simulink model "dPendDisEKF"  (Simulink 7.0)
settings: Solver=ode4  StartTime=0.0  StopTime=10  FixedStep=ts  RelTol=1e-3
InitFcn:
  | %dPendInit;
undefined symbols (not defined in the file): a, accel, B, b, c1, c2, d, evalJacobian, evalJacobMesr, g, l1, m1, m2, magnitude, p, P0, Qe, r1, r2, Re, ts, X0, x_0
libraries: simulink x4
settings Model: Creator=raje_ra  LastModifiedBy=raje_ra  BufferReuse=off
settings OptimizationCC: OptimizeBlockIOStorage=off  BufferReuse=off  ExpressionFolding=off  LocalBlockOutputs=off

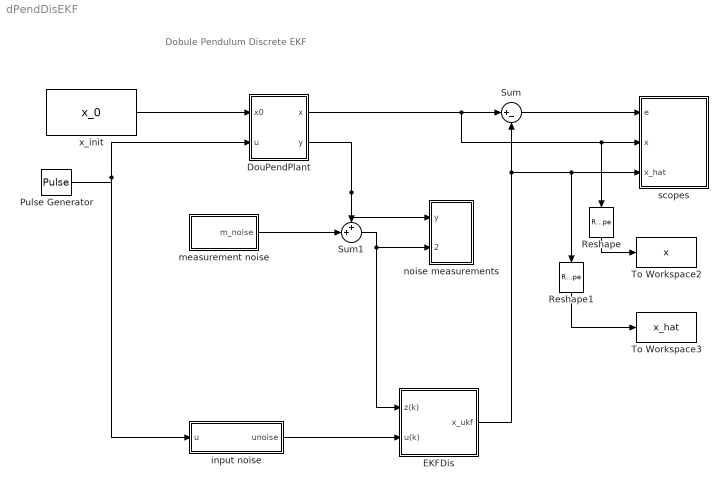
== system dPendDisEKF ==
  note: Dobule Pendulum Discrete EKF
  DouPendPlant : Subsystem
  EKFDis : Subsystem
  Pulse Generator : DiscretePulseGenerator  PulseType=Time based  Amplitude=0.01  Period=1  PulseWidth=50
  Reshape : Reshape  Orientation=down
  Reshape1 : Reshape  Orientation=down
  Sum : Sum  Inputs=|+-  OutDataType=sfix(16)  OutScaling=2^0
  Sum1 : Sum  Inputs=++|  OutDataType=sfix(16)  OutScaling=2^0
  To Workspace2 : ToWorkspace  VariableName=x  SampleTime=-1  SaveFormat=Structure With Time
  To Workspace3 : ToWorkspace  VariableName=x_hat  SampleTime=-1  SaveFormat=Structure With Time
  input noise : Subsystem
  measurement noise : Subsystem
  noise measurements : Subsystem
  scopes : Subsystem
  x_init : Constant  Value=x_0  VectorParams1D=off  OutDataType=sfix(16)  OutScaling=2^0
  wires:
  x_init/1 -> DouPendPlant/1(x0)
  DouPendPlant/1(x) -> Sum/1, scopes/2(x), Reshape/1
  EKFDis/1(x_ukf) -> Sum/2, scopes/3(x_hat), Reshape1/1
  Sum/1 -> scopes/1(e)
  Pulse Generator/1 -> DouPendPlant/2(u), input noise/1(u)
  DouPendPlant/2(y) -> Sum1/1, noise measurements/1(y)
  Sum1/1 -> EKFDis/1(z(k)), noise measurements/2(ynoise)
  measurement noise/1(m_noise) -> Sum1/2
  input noise/1(unoise) -> EKFDis/2(u(k))
  Reshape/1 -> To Workspace2/1
  Reshape1/1 -> To Workspace3/1

== system dPendDisEKF/DouPendPlant ==
  x0 : Inport
  u : Inport  Port=2
  F(x) : Subsystem
  Integrator1 : Integrator  InitialConditionSource=external  InitialCondition=[pi/3,-pi/3]'
  Measurements : Subsystem
  x : Outport  OutDataType=sfix(16)  OutScaling=2^0
  y : Outport  Port=2  OutDataType=sfix(16)  OutScaling=2^0
  wires:
  Measurements/1(y) -> y/1
  x0/1 -> Integrator1/2
  Integrator1/1 -> Measurements/1(x), F(x)/1(x), x/1  "x"
  F(x)/1(x_dot) -> Integrator1/1
  u/1 -> F(x)/2(u), Measurements/2(u)

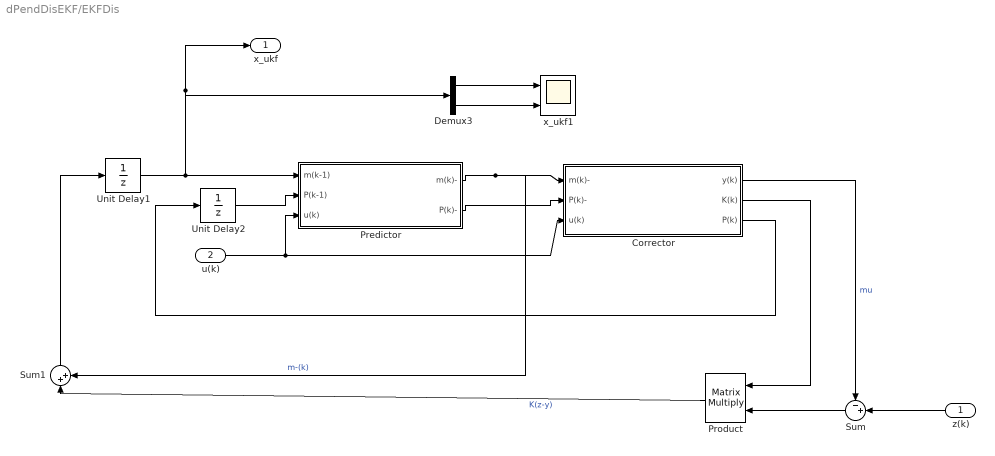
== system dPendDisEKF/EKFDis ==
  z(k) : Inport  Orientation=left
  u(k) : Inport  Port=2
  Corrector : Subsystem
  Demux3 : Demux  Outputs=2
  Predictor : Subsystem
  Product : Product  Orientation=left  Multiplication=Matrix(*)  OutDataType=sfix(16)  OutScaling=2^0  RndMeth=Zero
  Sum : Sum  Orientation=left  Inputs=-+|  OutDataType=sfix(16)  OutScaling=2^0
  Sum1 : Sum  Orientation=up  Inputs=|++  OutDataType=sfix(16)  OutScaling=2^0
  Unit Delay1 : UnitDelay  X0=X0  SampleTime=-1
  Unit Delay2 : UnitDelay  X0=P0  SampleTime=-1
  x_ukf1 : Scope  NumInputPorts=2
      settings: TimeRange=30  YMin=-15~-10  YMax=15~50  SaveName=ScopeData2
  x_ukf : Outport  OutDataType=sfix(16)  OutScaling=2^0
  wires:
  Corrector/3(P(k)) -> Unit Delay2/1
  Unit Delay2/1 -> Predictor/2(P(k-1))
  Product/1 -> Sum1/1  "K(z-y)"
  Sum/1 -> Product/2
  z(k)/1 -> Sum/2
  Corrector/2(K(k)) -> Product/1
  Corrector/1(y(k)) -> Sum/1  "mu"
  Predictor/2(P(k)-) -> Corrector/2(P(k)-)
  Predictor/1(m(k)-) -> Sum1/2, Corrector/1(m(k)-)  "m-(k)"
  Unit Delay1/1 -> Predictor/1(m(k-1)), x_ukf/1, Demux3/1
  Sum1/1 -> Unit Delay1/1
  Demux3/2 -> x_ukf1/2
  Demux3/1 -> x_ukf1/1
  u(k)/1 -> Predictor/3(u(k)), Corrector/3(u(k))

== system dPendDisEKF/input noise ==
  u : Inport
  Band-Limited White Noise : simulink/Sources/Band-Limited White Noise  SystemSampleTime=-1  Cov=[1e-6]  Ts=ts  seed=[23341]
  Sum2 : Sum  Inputs=++|  OutDataType=sfix(16)  OutScaling=2^0
  To Workspace2 : ToWorkspace  VariableName=Q_in  SampleTime=-1  SaveFormat=Array
  unoise : Outport
  wires:
  Band-Limited White Noise/1 -> Sum2/1, To Workspace2/1
  u/1 -> Sum2/2
  Sum2/1 -> unoise/1

== system dPendDisEKF/measurement noise ==
  Band-Limited White Noise - gyro : simulink/Sources/Band-Limited White Noise  SystemSampleTime=-1  Cov=[1e-7]  Ts=ts  seed=[23341]
  Band-Limited White Noise- q,dq : simulink/Sources/Band-Limited White Noise  SystemSampleTime=-1  Cov=[1e-9]  Ts=ts  seed=[23341]
  Band-Limited White Noise-IMU : simulink/Sources/Band-Limited White Noise  SystemSampleTime=-1  Cov=[1e-5]  Ts=ts  seed=[23341]
  Mux : Mux  Inputs=5
  To Workspace : ToWorkspace  VariableName=R_in  SampleTime=-1  SaveFormat=Array
  m_noise : Outport
  wires:
  Band-Limited White Noise- q,dq/1 -> Mux/1, Mux/2
  Mux/1 -> m_noise/1, To Workspace/1
  Band-Limited White Noise - gyro/1 -> Mux/3
  Band-Limited White Noise-IMU/1 -> Mux/4, Mux/5

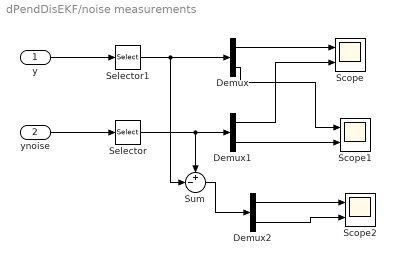
== system dPendDisEKF/noise measurements ==
  y : Inport
  ynoise : Inport  Port=2
  Demux : Demux  Outputs=2
  Demux1 : Demux  Outputs=2
  Demux2 : Demux  Outputs=2
  Scope : Scope  NumInputPorts=2
      settings: YMin=-60~-60  YMax=180~180
  Scope1 : Scope  NumInputPorts=2
      settings: YMin=-60~-60  YMax=180~180  SaveName=ScopeData5
  Scope2 : Scope  NumInputPorts=2
      settings: YMin=-60~-60  YMax=180~180  SaveName=ScopeData6
  Selector : Selector  InputPortWidth=5  IndexOptions=Index vector (dialog)  Indices=[4,5]  OutputSizes=1
  Selector1 : Selector  InputPortWidth=5  IndexOptions=Index vector (dialog)  Indices=[4,5]  OutputSizes=1
  Sum : Sum  Inputs=+-|  OutDataType=sfix(16)  OutScaling=2^0
  wires:
  y/1 -> Selector1/1
  ynoise/1 -> Selector/1
  Selector1/1 -> Demux/1, Sum/2
  Selector/1 -> Demux1/1, Sum/1
  Sum/1 -> Demux2/1
  Demux/1 -> Scope/1
  Demux1/1 -> Scope/2
  Demux/2 -> Scope1/1
  Demux1/2 -> Scope1/2
  Demux2/1 -> Scope2/1
  Demux2/2 -> Scope2/2

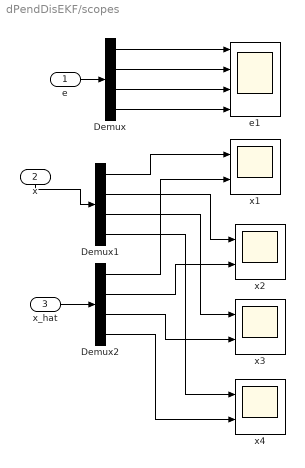
== system dPendDisEKF/scopes ==
  e : Inport
  x : Inport  Orientation=down  Port=2
  x_hat : Inport  Port=3
  Demux : Demux
  Demux1 : Demux
  Demux2 : Demux
  e1 : Scope  NumInputPorts=4
      settings: TickLabels=on  YMin=-30~-20~-120~-17.5  YMax=80~27.5~20~25
  x{1..4} (4 alike) : Scope  NumInputPorts=2
      x1 settings: TickLabels=on  YMin=-5~-5  YMax=14~22.5  SaveName=ScopeData3
      x2 settings: TickLabels=on  YMin=-11~-11  YMax=11~11  SaveName=ScopeData4
      x3 settings: TickLabels=on  YMin=-10~-10  YMax=27.5~27.5  SaveName=ScopeData7
      x4 settings: TickLabels=on  YMin=-40~-40  YMax=35~35  SaveName=ScopeData8
  wires:
  e/1 -> Demux/1
  x_hat/1 -> Demux2/1
  x/1 -> Demux1/1
  Demux2/4 -> x4/2
  Demux1/4 -> x4/1
  Demux2/3 -> x3/2
  Demux1/3 -> x3/1
  Demux2/2 -> x2/2
  Demux1/2 -> x2/1
  Demux2/1 -> x1/2
  Demux1/1 -> x1/1
  Demux/4 -> e1/4
  Demux/3 -> e1/3
  Demux/2 -> e1/2
  Demux/1 -> e1/1

== system dPendDisEKF/DouPendPlant/F(x) ==
  x : Inport
  u : Inport  Port=2
  Add : Sum  Inputs=+++  OutDataType=sfix(16)  OutScaling=2^-10
  Divide : Product  Inputs=/*  Multiplication=Matrix(*)  OutDataType=sfix(16)  OutScaling=2^-10
  Gain : Gain  Gain=diag([0,c1,0,c2])  Multiplication=Matrix(K*u)  ParameterDataType=sfix(16)  ParameterScaling=2^0  OutDataType=sfix(16)  OutScaling=2^0
  Gain1 : Gain  Gain=B  ParameterDataType=sfix(16)  ParameterScaling=2^0  OutDataType=sfix(16)  OutScaling=2^0
  M matrix : Subsystem
  h+g : Subsystem
  x_dot : Outport
  wires:
  Divide/1 -> x_dot/1
  M matrix/1(M) -> Divide/1
  Gain1/1 -> Add/3
  Add/1 -> Divide/2
  u/1 -> Gain1/1
  Gain/1 -> Add/2
  h+g/1(-(h+g)) -> Add/1
  x/1 -> Gain/1, h+g/1(x), M matrix/1(x)

== system dPendDisEKF/DouPendPlant/Measurements ==
  x : Inport
  u : Inport  Port=2
  Display : Display
  IMU : Subsystem
  Mux : Mux  Inputs=3
  Selector1 : Selector  InputPortWidth=4  IndexOptions=Index vector (dialog)  Indices=[3 4]  OutputSizes=1
  Selector2 : Selector  InputPortWidth=4  IndexOptions=Index vector (dialog)  Indices=[2 4]  OutputSizes=1
  Sum of Elements : Sum  Inputs=+  OutDataType=sfix(16)  OutScaling=2^-10
  y : Outport  OutDataType=sfix(16)  OutScaling=2^0
  wires:
  x/1 -> Selector1/1, Selector2/1, IMU/1(m(k)-)
  Selector1/1 -> Mux/1
  Mux/1 -> y/1, Display/1
  Selector2/1 -> Sum of Elements/1
  Sum of Elements/1 -> Mux/2  "(dq_1+dq_2)"
  u/1 -> IMU/2(u(k))
  IMU/1(acc) -> Mux/3

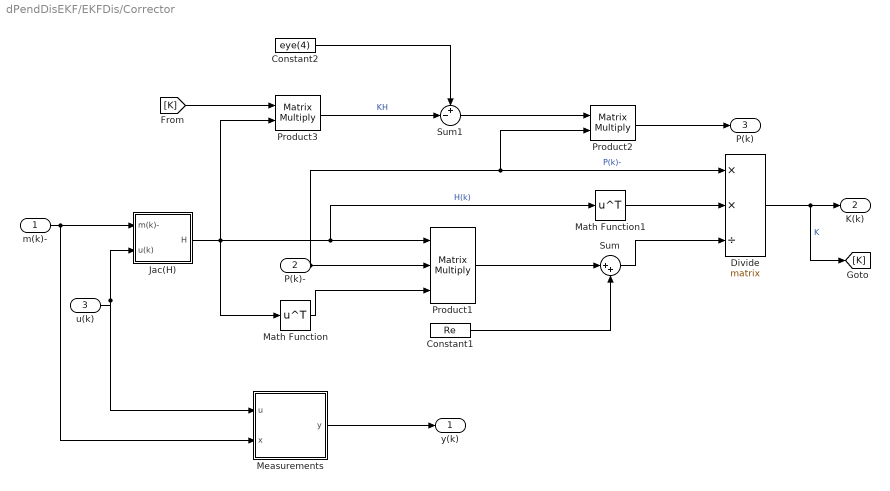
== system dPendDisEKF/EKFDis/Corrector ==
  m(k)- : Inport
  P(k)- : Inport  Port=2
  u(k) : Inport  Port=3
  Constant1 : Constant  Value=Re  OutDataType=sfix(16)  OutScaling=2^0
  Constant2 : Constant  Value=eye(4)  VectorParams1D=off  OutDataType=sfix(16)  OutScaling=2^0
  Divide : Product  Inputs=**/  Multiplication=Matrix(*)  OutDataType=sfix(16)  OutScaling=2^-10
  Jac(H) : Subsystem
  Math Function : Math  Operator=transpose  OutDataType=sfix(16)  OutScaling=2^0  SaturateOnIntegerOverflow=on
  Math Function1 : Math  Operator=transpose  OutDataType=sfix(16)  OutScaling=2^0  SaturateOnIntegerOverflow=on
  Measurements : Subsystem
  Product1 : Product  Inputs=3  Multiplication=Matrix(*)  OutDataType=sfix(16)  OutScaling=2^0  RndMeth=Zero
  Product2 : Product  Multiplication=Matrix(*)  OutDataType=sfix(16)  OutScaling=2^0  RndMeth=Zero
  Product3 : Product  Multiplication=Matrix(*)  OutDataType=sfix(16)  OutScaling=2^0  RndMeth=Zero
  Sum : Sum  Inputs=|++  OutDataType=sfix(16)  OutScaling=2^0
  Sum1 : Sum  Inputs=+-|  OutDataType=sfix(16)  OutScaling=2^0
  y(k) : Outport
  K(k) : Outport  Port=2
  P(k) : Outport  Port=3
  wires:
  Constant1/1 -> Sum/2
  Product1/1 -> Sum/1
  m(k)-/1 -> Jac(H)/1(m(k)-), Measurements/2(x)
  u(k)/1 -> Jac(H)/2(u(k)), Measurements/1(u)
  Jac(H)/1(H) -> Math Function/1, Product3/2, Product1/1, Math Function1/1  "H(k)"
  P(k)-/1 -> Product1/2, Divide/1, Product2/2  "P(k)-"
  Math Function/1 -> Product1/3
  Sum/1 -> Divide/3
  Divide/1 -> K(k)/1, [K]  "K"
  [K] -> Product3/1
  Constant2/1 -> Sum1/1
  Product3/1 -> Sum1/2  "KH"
  Sum1/1 -> Product2/1
  Product2/1 -> P(k)/1
  Measurements/1(y) -> y(k)/1
  Math Function1/1 -> Divide/2

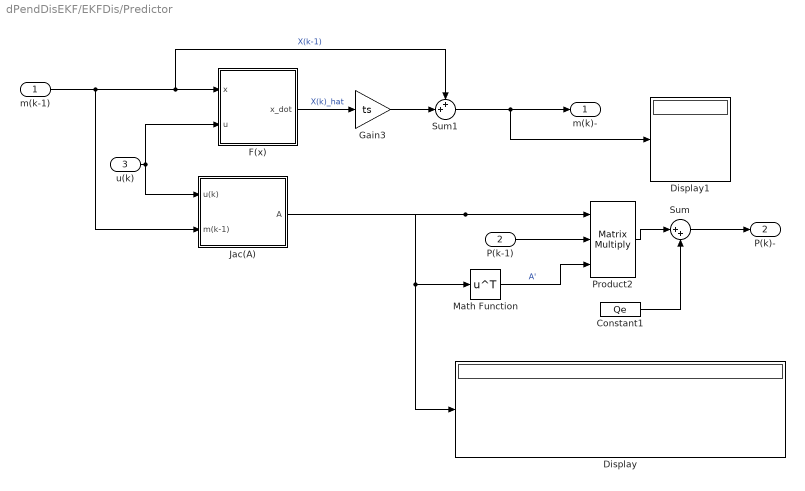
== system dPendDisEKF/EKFDis/Predictor ==
  m(k-1) : Inport
  P(k-1) : Inport  Port=2
  u(k) : Inport  Port=3
  Constant1 : Constant  Value=Qe  OutDataType=sfix(16)  OutScaling=2^0
  Display : Display
  Display1 : Display
  F(x) : Subsystem
  Gain3 : Gain  Gain=ts  ParameterDataType=sfix(16)  ParameterScaling=2^0  OutDataType=sfix(16)  OutScaling=2^0
  Jac(A) : Subsystem
  Math Function : Math  Operator=transpose  OutDataType=sfix(16)  OutScaling=2^0  SaturateOnIntegerOverflow=on
  Product2 : Product  Inputs=3  Multiplication=Matrix(*)  OutDataType=sfix(16)  OutScaling=2^0  RndMeth=Zero
  Sum : Sum  Inputs=|++  OutDataType=sfix(16)  OutScaling=2^0
  Sum1 : Sum  Inputs=++|  OutDataType=sfix(16)  OutScaling=2^0
  m(k)- : Outport
  P(k)- : Outport  Port=2
  wires:
  Sum/1 -> P(k)-/1
  Constant1/1 -> Sum/2
  Product2/1 -> Sum/1
  m(k-1)/1 -> Jac(A)/2(m(k-1)), F(x)/1(x), Sum1/1  "X(k-1)"
  u(k)/1 -> Jac(A)/1(u(k)), F(x)/2(u)
  F(x)/1(x_dot) -> Gain3/1  "X(k)_hat"
  Jac(A)/1(A) -> Product2/1, Math Function/1, Display/1
  P(k-1)/1 -> Product2/2
  Math Function/1 -> Product2/3  "A'"
  Gain3/1 -> Sum1/2
  Sum1/1 -> m(k)-/1, Display1/1

== system dPendDisEKF/DouPendPlant/F(x)/M matrix ==
  x : Inport
  M1 : Constant  Value=[1,0,0,0]  VectorParams1D=off  OutDataType=sfix(16)  OutScaling=2^0
  M2 : Subsystem
  M3 : Constant  Value=[0,0,1,0]  VectorParams1D=off  OutDataType=sfix(16)  OutScaling=2^0
  M4 : Subsystem
  Matrix Concatenate : Concatenate  NumInputs=4  Mode=Multidimensional array
  Selector : Selector  InputPortWidth=4  IndexOptions=Index vector (dialog)  Indices=[3]  OutputSizes=1
  M : Outport
  wires:
  Matrix Concatenate/1 -> M/1
  x/1 -> Selector/1
  M4/1(Out) -> Matrix Concatenate/4
  M3/1 -> Matrix Concatenate/3
  M2/1(Out1) -> Matrix Concatenate/2
  M1/1 -> Matrix Concatenate/1
  Selector/1 -> M4/1(x3), M2/1(x3)  "x3"

== system dPendDisEKF/DouPendPlant/F(x)/h+g ==
  x : Inport
  Selector : Selector  InputPortWidth=4  IndexOptions=Index vector (dialog)  Indices=[2]  OutputSizes=1
  Selector1 : Selector  InputPortWidth=4  IndexOptions=Index vector (dialog)  Indices=[4]  OutputSizes=1
  Vector Concatenate : Concatenate  NumInputs=4  Mode=Vector
  h+g(2) : Subsystem
  h+g(4) : Subsystem
  -(h+g) : Outport
  wires:
  Vector Concatenate/1 -> -(h+g)/1
  h+g(4)/1(-F(2)) -> Vector Concatenate/4
  Selector1/1 -> Vector Concatenate/3
  h+g(2)/1(-F(1)) -> Vector Concatenate/2
  Selector/1 -> Vector Concatenate/1  "x2"
  x/1 -> h+g(4)/1(x), Selector1/1, h+g(2)/1(x), Selector/1

== system dPendDisEKF/DouPendPlant/Measurements/IMU ==
  m(k)- : Inport
  u(k) : Inport  Port=2
  Mux : Mux  Inputs=2
  Transpose : Math  Operator=transpose  OutDataType=sfix(16)  OutScaling=2^0  SaturateOnIntegerOverflow=on
  acceleration : MATLABFcn  MATLABFcn=accel(u,p)  Output1D=off
  acc : Outport
  wires:
  Mux/1 -> Transpose/1
  Transpose/1 -> acceleration/1
  m(k)-/1 -> Mux/1
  acceleration/1 -> acc/1  "acc"
  u(k)/1 -> Mux/2

== system dPendDisEKF/EKFDis/Corrector/Jac(H) ==
  m(k)- : Inport
  u(k) : Inport  Port=2
  Display : Display
  Display1 : Display
  Jacob Mesr : MATLABFcn  MATLABFcn=evalJacobMesr(u,p)  Output1D=off
  Mux : Mux  Inputs=2
  Transpose : Math  Operator=transpose  OutDataType=sfix(16)  OutScaling=2^0  SaturateOnIntegerOverflow=on
  H : Outport
  wires:
  Mux/1 -> Transpose/1, Display1/1
  Transpose/1 -> Jacob Mesr/1
  m(k)-/1 -> Mux/1
  Jacob Mesr/1 -> H/1, Display/1  "h"
  u(k)/1 -> Mux/2

== system dPendDisEKF/EKFDis/Corrector/Measurements ==
  u : Inport
  x : Inport  Port=2
  IMU : Subsystem
  Mux : Mux  Inputs=3
  Selector1 : Selector  InputPortWidth=4  IndexOptions=Index vector (dialog)  Indices=[3 4]  OutputSizes=1
  Selector2 : Selector  InputPortWidth=4  IndexOptions=Index vector (dialog)  Indices=[2 4]  OutputSizes=1
  Sum of Elements : Sum  Inputs=+  OutDataType=sfix(16)  OutScaling=2^-10
  y : Outport  OutDataType=sfix(16)  OutScaling=2^0
  wires:
  x/1 -> Selector1/1, Selector2/1, IMU/1(m(k)-)
  Selector1/1 -> Mux/1
  Mux/1 -> y/1
  Selector2/1 -> Sum of Elements/1
  Sum of Elements/1 -> Mux/2  "(dq_1+dq_2)"
  u/1 -> IMU/2(u(k))
  IMU/1(acc) -> Mux/3

== system dPendDisEKF/EKFDis/Predictor/F(x) ==
  x : Inport
  u : Inport  Port=2
  Add : Sum  Inputs=+++  OutDataType=sfix(16)  OutScaling=2^-10
  Divide : Product  Inputs=/*  Multiplication=Matrix(*)  OutDataType=sfix(16)  OutScaling=2^-10
  Gain : Gain  Gain=diag([0,c1,0,c2])  Multiplication=Matrix(K*u)  ParameterDataType=sfix(16)  ParameterScaling=2^0  OutDataType=sfix(16)  OutScaling=2^0
  Gain1 : Gain  Gain=B  ParameterDataType=sfix(16)  ParameterScaling=2^0  OutDataType=sfix(16)  OutScaling=2^0
  M matrix : Subsystem
  h+g : Subsystem
  x_dot : Outport
  wires:
  Divide/1 -> x_dot/1
  M matrix/1(M) -> Divide/1
  Gain1/1 -> Add/3
  Add/1 -> Divide/2
  u/1 -> Gain1/1
  Gain/1 -> Add/2
  h+g/1(-(h+g)) -> Add/1
  x/1 -> h+g/1(x), Gain/1, M matrix/1(x)

== system dPendDisEKF/EKFDis/Predictor/Jac(A) ==
  u(k) : Inport
  m(k-1) : Inport  Port=2
  Display : Display
  Display1 : Display
  MATLAB Fcn : MATLABFcn  MATLABFcn=evalJacobian(u,p)  Output1D=off
  Math Function1 : Math  Operator=transpose  OutDataType=sfix(16)  OutScaling=2^0  SaturateOnIntegerOverflow=on
  Mux : Mux  Inputs=2
  A : Outport
  wires:
  Math Function1/1 -> MATLAB Fcn/1, Display1/1
  MATLAB Fcn/1 -> A/1, Display/1  "A"
  m(k-1)/1 -> Mux/1
  u(k)/1 -> Mux/2
  Mux/1 -> Math Function1/1

== system dPendDisEKF/DouPendPlant/F(x)/M matrix/M2 ==
  x3 : Inport
  M21 : Constant  Value=0  VectorParams1D=off  OutDataType=sfix(16)  OutScaling=2^0
  M22 : Subsystem
  M23 : Constant  Value=0  VectorParams1D=off  OutDataType=sfix(16)  OutScaling=2^0
  M24 : Subsystem
  Math Function : Math  Operator=transpose  OutDataType=sfix(16)  OutScaling=2^0  SaturateOnIntegerOverflow=on
  Vector Concatenate : Concatenate  NumInputs=4  Mode=Vector
  Out1 : Outport
  wires:
  Math Function/1 -> Out1/1
  Vector Concatenate/1 -> Math Function/1
  M24/1(M24) -> Vector Concatenate/4
  M23/1 -> Vector Concatenate/3
  M22/1(M22) -> Vector Concatenate/2
  M21/1 -> Vector Concatenate/1
  x3/1 -> M24/1(x3), M22/1(x3)

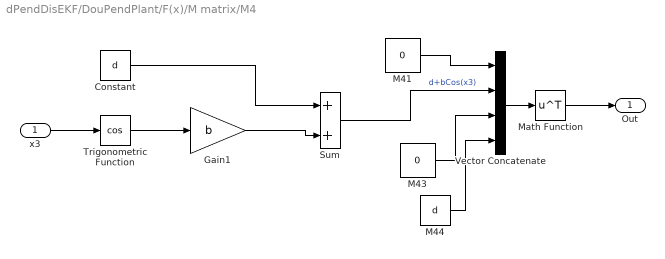
== system dPendDisEKF/DouPendPlant/F(x)/M matrix/M4 ==
  x3 : Inport
  Constant : Constant  Value=d  OutDataType=sfix(16)  OutScaling=2^0
  Gain1 : Gain  Gain=b  ParameterDataType=sfix(16)  ParameterScaling=2^0  OutDataType=sfix(16)  OutScaling=2^0
  M41 : Constant  Value=0  VectorParams1D=off  OutDataType=sfix(16)  OutScaling=2^0
  M43 : Constant  Value=0  VectorParams1D=off  OutDataType=sfix(16)  OutScaling=2^0
  M44 : Constant  Value=d  OutDataType=sfix(16)  OutScaling=2^0
  Math Function : Math  Operator=transpose  OutDataType=sfix(16)  OutScaling=2^0  SaturateOnIntegerOverflow=on
  Sum : Sum  OutDataType=sfix(16)  OutScaling=2^0
  Trigonometric Function : Trigonometry  Operator=cos
  Vector Concatenate : Concatenate  NumInputs=4  Mode=Vector
  Out : Outport
  wires:
  Constant/1 -> Sum/1
  Math Function/1 -> Out/1
  Vector Concatenate/1 -> Math Function/1
  M43/1 -> Vector Concatenate/3
  M44/1 -> Vector Concatenate/4
  Sum/1 -> Vector Concatenate/2  "d+bCos(x3)"
  M41/1 -> Vector Concatenate/1
  Trigonometric Function/1 -> Gain1/1
  Gain1/1 -> Sum/2
  x3/1 -> Trigonometric Function/1

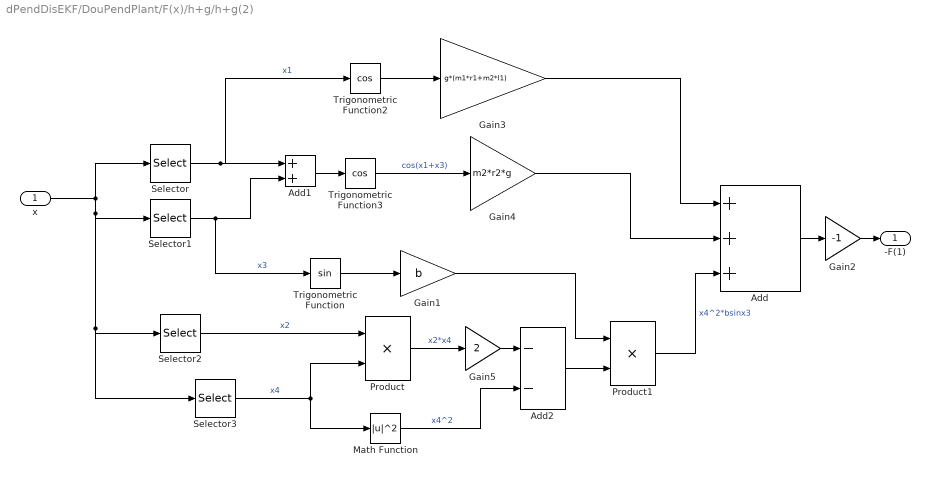
== system dPendDisEKF/DouPendPlant/F(x)/h+g/h+g(2) ==
  x : Inport
  Add : Sum  Inputs=+++  OutDataType=sfix(16)  OutScaling=2^-10
  Add1 : Sum  OutDataType=sfix(16)  OutScaling=2^-10
  Add2 : Sum  Inputs=--  OutDataType=sfix(16)  OutScaling=2^-10
  Gain1 : Gain  Gain=b  ParameterDataType=sfix(16)  ParameterScaling=2^0  OutDataType=sfix(16)  OutScaling=2^0
  Gain2 : Gain  Gain=-1  ParameterDataType=sfix(16)  ParameterScaling=2^0  OutDataType=sfix(16)  OutScaling=2^0
  Gain3 : Gain  Gain=g*(m1*r1+m2*l1)  ParameterDataType=sfix(16)  ParameterScaling=2^0  OutDataType=sfix(16)  OutScaling=2^0
  Gain4 : Gain  Gain=m2*r2*g  ParameterDataType=sfix(16)  ParameterScaling=2^0  OutDataType=sfix(16)  OutScaling=2^0
  Gain5 : Gain  Gain=2  ParameterDataType=sfix(16)  ParameterScaling=2^0  OutDataType=sfix(16)  OutScaling=2^0
  Math Function : Math  Operator=magnitude^2  OutDataType=sfix(16)  OutScaling=2^0  SaturateOnIntegerOverflow=on
  Product : Product  OutDataType=sfix(16)  OutScaling=2^0  RndMeth=Zero
  Product1 : Product  OutDataType=sfix(16)  OutScaling=2^0  RndMeth=Zero
  Selector : Selector  InputPortWidth=4  IndexOptions=Index vector (dialog)  Indices=[1]  OutputSizes=1
  Selector1 : Selector  InputPortWidth=4  IndexOptions=Index vector (dialog)  Indices=[3]  OutputSizes=1
  Selector2 : Selector  InputPortWidth=4  IndexOptions=Index vector (dialog)  Indices=[2]  OutputSizes=1
  Selector3 : Selector  InputPortWidth=4  IndexOptions=Index vector (dialog)  Indices=[4]  OutputSizes=1
  Trigonometric Function : Trigonometry
  Trigonometric Function2 : Trigonometry  Operator=cos
  Trigonometric Function3 : Trigonometry  Operator=cos
  -F(1) : Outport  OutDataType=sfix(16)  OutScaling=2^0
  wires:
  Gain2/1 -> -F(1)/1
  Gain1/1 -> Product1/1
  Add2/1 -> Product1/2
  Gain5/1 -> Add2/1
  Product/1 -> Gain5/1  "x2*x4"
  Math Function/1 -> Add2/2  "x4^2"
  Selector2/1 -> Product/1  "x2"
  Selector3/1 -> Math Function/1, Product/2  "x4"
  x/1 -> Selector3/1, Selector2/1, Selector1/1, Selector/1
  Add/1 -> Gain2/1
  Product1/1 -> Add/3  "x4^2*bsinx3"
  Gain4/1 -> Add/2
  Add1/1 -> Trigonometric Function3/1
  Trigonometric Function3/1 -> Gain4/1  "cos(x1+x3)"
  Gain3/1 -> Add/1
  Trigonometric Function2/1 -> Gain3/1
  Selector/1 -> Trigonometric Function2/1, Add1/1  "x1"
  Selector1/1 -> Trigonometric Function/1, Add1/2  "x3"
  Trigonometric Function/1 -> Gain1/1

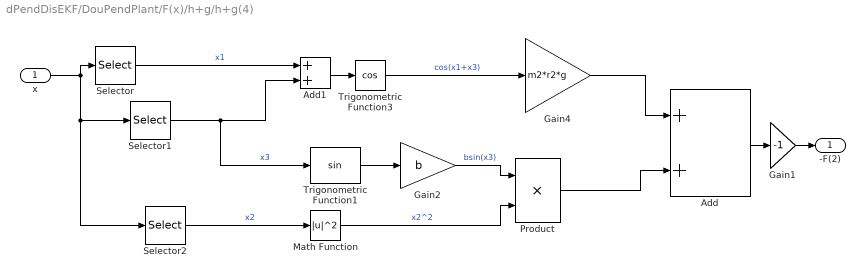
== system dPendDisEKF/DouPendPlant/F(x)/h+g/h+g(4) ==
  x : Inport
  Add : Sum  OutDataType=sfix(16)  OutScaling=2^-10
  Add1 : Sum  OutDataType=sfix(16)  OutScaling=2^-10
  Gain1 : Gain  Gain=-1  ParameterDataType=sfix(16)  ParameterScaling=2^0  OutDataType=sfix(16)  OutScaling=2^0
  Gain2 : Gain  Gain=b  ParameterDataType=sfix(16)  ParameterScaling=2^0  OutDataType=sfix(16)  OutScaling=2^0
  Gain4 : Gain  Gain=m2*r2*g  ParameterDataType=sfix(16)  ParameterScaling=2^0  OutDataType=sfix(16)  OutScaling=2^0
  Math Function : Math  Operator=magnitude^2  OutDataType=sfix(16)  OutScaling=2^0  SaturateOnIntegerOverflow=on
  Product : Product  OutDataType=sfix(16)  OutScaling=2^0  RndMeth=Zero
  Selector : Selector  InputPortWidth=4  IndexOptions=Index vector (dialog)  Indices=[1]  OutputSizes=1
  Selector1 : Selector  InputPortWidth=4  IndexOptions=Index vector (dialog)  Indices=[3]  OutputSizes=1
  Selector2 : Selector  InputPortWidth=4  IndexOptions=Index vector (dialog)  Indices=[2]  OutputSizes=1
  Trigonometric Function1 : Trigonometry
  Trigonometric Function3 : Trigonometry  Operator=cos
  -F(2) : Outport  OutDataType=sfix(16)  OutScaling=2^0
  wires:
  Gain1/1 -> -F(2)/1
  Math Function/1 -> Product/2  "x2^2"
  Gain2/1 -> Product/1  "bsin(x3)"
  Add/1 -> Gain1/1
  Add1/1 -> Trigonometric Function3/1
  Trigonometric Function3/1 -> Gain4/1  "cos(x1+x3)"
  Selector/1 -> Add1/1  "x1"
  Selector1/1 -> Add1/2, Trigonometric Function1/1  "x3"
  Trigonometric Function1/1 -> Gain2/1
  x/1 -> Selector2/1, Selector1/1, Selector/1
  Gain4/1 -> Add/1
  Product/1 -> Add/2
  Selector2/1 -> Math Function/1  "x2"

== system dPendDisEKF/EKFDis/Corrector/Measurements/IMU ==
  m(k)- : Inport
  u(k) : Inport  Port=2
  Mux : Mux  Inputs=2
  Transpose : Math  Operator=transpose  OutDataType=sfix(16)  OutScaling=2^0  SaturateOnIntegerOverflow=on
  accleration : MATLABFcn  MATLABFcn=accel(u,p)  Output1D=off
  acc : Outport
  wires:
  Mux/1 -> Transpose/1
  Transpose/1 -> accleration/1
  m(k)-/1 -> Mux/1
  accleration/1 -> acc/1  "acc"
  u(k)/1 -> Mux/2

== system dPendDisEKF/EKFDis/Predictor/F(x)/M matrix ==
  x : Inport
  M1 : Constant  Value=[1,0,0,0]  VectorParams1D=off  OutDataType=sfix(16)  OutScaling=2^0
  M2 : Subsystem
  M3 : Constant  Value=[0,0,1,0]  VectorParams1D=off  OutDataType=sfix(16)  OutScaling=2^0
  M4 : Subsystem
  Matrix Concatenate : Concatenate  NumInputs=4  Mode=Multidimensional array
  Selector : Selector  InputPortWidth=4  IndexOptions=Index vector (dialog)  Indices=[3]  OutputSizes=1
  M : Outport
  wires:
  Matrix Concatenate/1 -> M/1
  x/1 -> Selector/1
  M4/1(Out) -> Matrix Concatenate/4
  M3/1 -> Matrix Concatenate/3
  M2/1(Out1) -> Matrix Concatenate/2
  M1/1 -> Matrix Concatenate/1
  Selector/1 -> M4/1(x3), M2/1(x3)  "x3"

== system dPendDisEKF/EKFDis/Predictor/F(x)/h+g ==
  x : Inport
  Selector : Selector  InputPortWidth=4  IndexOptions=Index vector (dialog)  Indices=[2]  OutputSizes=1
  Selector1 : Selector  InputPortWidth=4  IndexOptions=Index vector (dialog)  Indices=[4]  OutputSizes=1
  Vector Concatenate : Concatenate  NumInputs=4  Mode=Vector
  h+g(2) : Subsystem
  h+g(4) : Subsystem
  -(h+g) : Outport
  wires:
  Vector Concatenate/1 -> -(h+g)/1
  h+g(4)/1(-F(2)) -> Vector Concatenate/4
  Selector1/1 -> Vector Concatenate/3
  h+g(2)/1(-F(1)) -> Vector Concatenate/2
  Selector/1 -> Vector Concatenate/1  "x2"
  x/1 -> h+g(4)/1(x), Selector1/1, h+g(2)/1(x), Selector/1

== system dPendDisEKF/DouPendPlant/F(x)/M matrix/M2/M22 ==
  x3 : Inport
  Constant : Constant  Value=a  OutDataType=sfix(16)  OutScaling=2^0
  Gain1 : Gain  Gain=2*b  ParameterDataType=sfix(16)  ParameterScaling=2^0  OutDataType=sfix(16)  OutScaling=2^0
  Sum : Sum  OutDataType=sfix(16)  OutScaling=2^0
  Trigonometric Function : Trigonometry  Operator=cos
  M22 : Outport
  wires:
  Constant/1 -> Sum/1
  Trigonometric Function/1 -> Gain1/1
  Gain1/1 -> Sum/2
  Sum/1 -> M22/1  "a+2bCos(x3)"
  x3/1 -> Trigonometric Function/1

== system dPendDisEKF/DouPendPlant/F(x)/M matrix/M2/M24 ==
  x3 : Inport
  Constant : Constant  Value=d  OutDataType=sfix(16)  OutScaling=2^0
  Gain1 : Gain  Gain=b  ParameterDataType=sfix(16)  ParameterScaling=2^0  OutDataType=sfix(16)  OutScaling=2^0
  Sum : Sum  OutDataType=sfix(16)  OutScaling=2^0
  Trigonometric Function : Trigonometry  Operator=cos
  M24 : Outport
  wires:
  Constant/1 -> Sum/1
  x3/1 -> Trigonometric Function/1
  Sum/1 -> M24/1  "d+bCos(x3)"
  Gain1/1 -> Sum/2
  Trigonometric Function/1 -> Gain1/1

== system dPendDisEKF/EKFDis/Predictor/F(x)/M matrix/M2 ==
  x3 : Inport
  M21 : Constant  Value=0  VectorParams1D=off  OutDataType=sfix(16)  OutScaling=2^0
  M22 : Subsystem
  M23 : Constant  Value=0  VectorParams1D=off  OutDataType=sfix(16)  OutScaling=2^0
  M24 : Subsystem
  Math Function : Math  Operator=transpose  OutDataType=sfix(16)  OutScaling=2^0  SaturateOnIntegerOverflow=on
  Vector Concatenate : Concatenate  NumInputs=4  Mode=Vector
  Out1 : Outport
  wires:
  Math Function/1 -> Out1/1
  Vector Concatenate/1 -> Math Function/1
  M24/1(M24) -> Vector Concatenate/4
  M23/1 -> Vector Concatenate/3
  M22/1(M22) -> Vector Concatenate/2
  M21/1 -> Vector Concatenate/1
  x3/1 -> M24/1(x3), M22/1(x3)

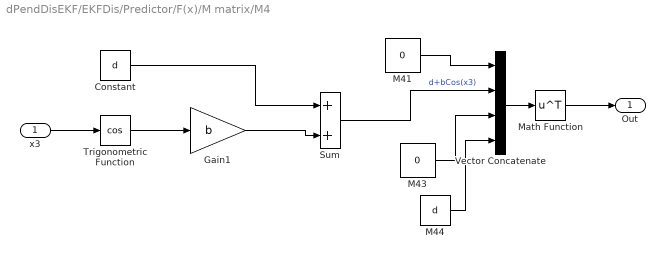
== system dPendDisEKF/EKFDis/Predictor/F(x)/M matrix/M4 ==
  x3 : Inport
  Constant : Constant  Value=d  OutDataType=sfix(16)  OutScaling=2^0
  Gain1 : Gain  Gain=b  ParameterDataType=sfix(16)  ParameterScaling=2^0  OutDataType=sfix(16)  OutScaling=2^0
  M41 : Constant  Value=0  VectorParams1D=off  OutDataType=sfix(16)  OutScaling=2^0
  M43 : Constant  Value=0  VectorParams1D=off  OutDataType=sfix(16)  OutScaling=2^0
  M44 : Constant  Value=d  OutDataType=sfix(16)  OutScaling=2^0
  Math Function : Math  Operator=transpose  OutDataType=sfix(16)  OutScaling=2^0  SaturateOnIntegerOverflow=on
  Sum : Sum  OutDataType=sfix(16)  OutScaling=2^0
  Trigonometric Function : Trigonometry  Operator=cos
  Vector Concatenate : Concatenate  NumInputs=4  Mode=Vector
  Out : Outport
  wires:
  Constant/1 -> Sum/1
  Math Function/1 -> Out/1
  Vector Concatenate/1 -> Math Function/1
  M43/1 -> Vector Concatenate/3
  M44/1 -> Vector Concatenate/4
  Sum/1 -> Vector Concatenate/2  "d+bCos(x3)"
  M41/1 -> Vector Concatenate/1
  Trigonometric Function/1 -> Gain1/1
  Gain1/1 -> Sum/2
  x3/1 -> Trigonometric Function/1

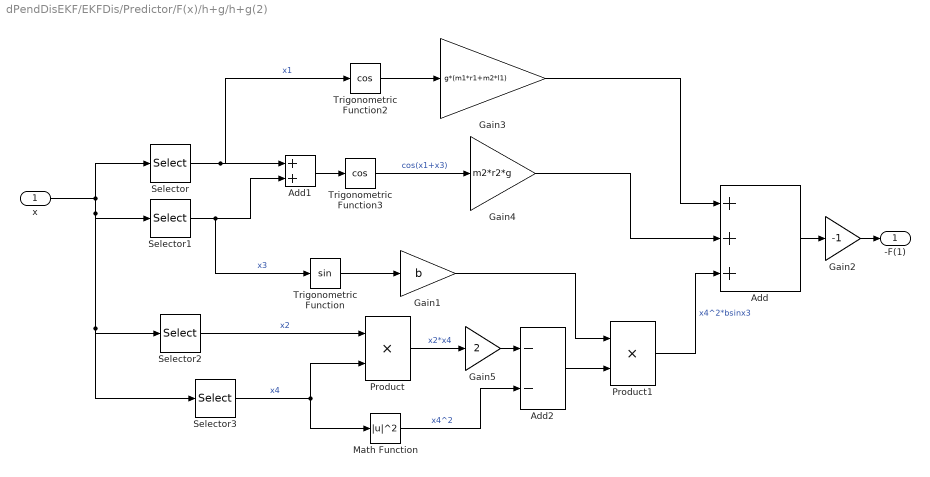
== system dPendDisEKF/EKFDis/Predictor/F(x)/h+g/h+g(2) ==
  x : Inport
  Add : Sum  Inputs=+++  OutDataType=sfix(16)  OutScaling=2^-10
  Add1 : Sum  OutDataType=sfix(16)  OutScaling=2^-10
  Add2 : Sum  Inputs=--  OutDataType=sfix(16)  OutScaling=2^-10
  Gain1 : Gain  Gain=b  ParameterDataType=sfix(16)  ParameterScaling=2^0  OutDataType=sfix(16)  OutScaling=2^0
  Gain2 : Gain  Gain=-1  ParameterDataType=sfix(16)  ParameterScaling=2^0  OutDataType=sfix(16)  OutScaling=2^0
  Gain3 : Gain  Gain=g*(m1*r1+m2*l1)  ParameterDataType=sfix(16)  ParameterScaling=2^0  OutDataType=sfix(16)  OutScaling=2^0
  Gain4 : Gain  Gain=m2*r2*g  ParameterDataType=sfix(16)  ParameterScaling=2^0  OutDataType=sfix(16)  OutScaling=2^0
  Gain5 : Gain  Gain=2  ParameterDataType=sfix(16)  ParameterScaling=2^0  OutDataType=sfix(16)  OutScaling=2^0
  Math Function : Math  Operator=magnitude^2  OutDataType=sfix(16)  OutScaling=2^0  SaturateOnIntegerOverflow=on
  Product : Product  OutDataType=sfix(16)  OutScaling=2^0  RndMeth=Zero
  Product1 : Product  OutDataType=sfix(16)  OutScaling=2^0  RndMeth=Zero
  Selector : Selector  InputPortWidth=4  IndexOptions=Index vector (dialog)  Indices=[1]  OutputSizes=1
  Selector1 : Selector  InputPortWidth=4  IndexOptions=Index vector (dialog)  Indices=[3]  OutputSizes=1
  Selector2 : Selector  InputPortWidth=4  IndexOptions=Index vector (dialog)  Indices=[2]  OutputSizes=1
  Selector3 : Selector  InputPortWidth=4  IndexOptions=Index vector (dialog)  Indices=[4]  OutputSizes=1
  Trigonometric Function : Trigonometry
  Trigonometric Function2 : Trigonometry  Operator=cos
  Trigonometric Function3 : Trigonometry  Operator=cos
  -F(1) : Outport  OutDataType=sfix(16)  OutScaling=2^0
  wires:
  Gain2/1 -> -F(1)/1
  Gain1/1 -> Product1/1
  Add2/1 -> Product1/2
  Gain5/1 -> Add2/1
  Product/1 -> Gain5/1  "x2*x4"
  Math Function/1 -> Add2/2  "x4^2"
  Selector2/1 -> Product/1  "x2"
  Selector3/1 -> Math Function/1, Product/2  "x4"
  x/1 -> Selector3/1, Selector2/1, Selector1/1, Selector/1
  Add/1 -> Gain2/1
  Product1/1 -> Add/3  "x4^2*bsinx3"
  Gain4/1 -> Add/2
  Add1/1 -> Trigonometric Function3/1
  Trigonometric Function3/1 -> Gain4/1  "cos(x1+x3)"
  Gain3/1 -> Add/1
  Trigonometric Function2/1 -> Gain3/1
  Selector/1 -> Trigonometric Function2/1, Add1/1  "x1"
  Selector1/1 -> Trigonometric Function/1, Add1/2  "x3"
  Trigonometric Function/1 -> Gain1/1

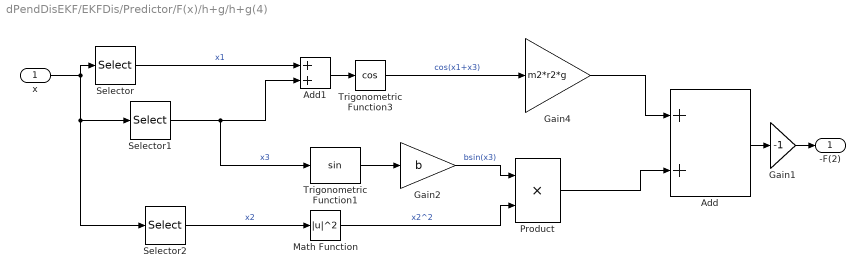
== system dPendDisEKF/EKFDis/Predictor/F(x)/h+g/h+g(4) ==
  x : Inport
  Add : Sum  OutDataType=sfix(16)  OutScaling=2^-10
  Add1 : Sum  OutDataType=sfix(16)  OutScaling=2^-10
  Gain1 : Gain  Gain=-1  ParameterDataType=sfix(16)  ParameterScaling=2^0  OutDataType=sfix(16)  OutScaling=2^0
  Gain2 : Gain  Gain=b  ParameterDataType=sfix(16)  ParameterScaling=2^0  OutDataType=sfix(16)  OutScaling=2^0
  Gain4 : Gain  Gain=m2*r2*g  ParameterDataType=sfix(16)  ParameterScaling=2^0  OutDataType=sfix(16)  OutScaling=2^0
  Math Function : Math  Operator=magnitude^2  OutDataType=sfix(16)  OutScaling=2^0  SaturateOnIntegerOverflow=on
  Product : Product  OutDataType=sfix(16)  OutScaling=2^0  RndMeth=Zero
  Selector : Selector  InputPortWidth=4  IndexOptions=Index vector (dialog)  Indices=[1]  OutputSizes=1
  Selector1 : Selector  InputPortWidth=4  IndexOptions=Index vector (dialog)  Indices=[3]  OutputSizes=1
  Selector2 : Selector  InputPortWidth=4  IndexOptions=Index vector (dialog)  Indices=[2]  OutputSizes=1
  Trigonometric Function1 : Trigonometry
  Trigonometric Function3 : Trigonometry  Operator=cos
  -F(2) : Outport  OutDataType=sfix(16)  OutScaling=2^0
  wires:
  Gain1/1 -> -F(2)/1
  Math Function/1 -> Product/2  "x2^2"
  Gain2/1 -> Product/1  "bsin(x3)"
  Add/1 -> Gain1/1
  Add1/1 -> Trigonometric Function3/1
  Trigonometric Function3/1 -> Gain4/1  "cos(x1+x3)"
  Selector/1 -> Add1/1  "x1"
  Selector1/1 -> Add1/2, Trigonometric Function1/1  "x3"
  Trigonometric Function1/1 -> Gain2/1
  x/1 -> Selector2/1, Selector1/1, Selector/1
  Gain4/1 -> Add/1
  Product/1 -> Add/2
  Selector2/1 -> Math Function/1  "x2"

== system dPendDisEKF/EKFDis/Predictor/F(x)/M matrix/M2/M22 ==
  x3 : Inport
  Constant : Constant  Value=a  OutDataType=sfix(16)  OutScaling=2^0
  Gain1 : Gain  Gain=2*b  ParameterDataType=sfix(16)  ParameterScaling=2^0  OutDataType=sfix(16)  OutScaling=2^0
  Sum : Sum  OutDataType=sfix(16)  OutScaling=2^0
  Trigonometric Function : Trigonometry  Operator=cos
  M22 : Outport
  wires:
  Constant/1 -> Sum/1
  Trigonometric Function/1 -> Gain1/1
  Gain1/1 -> Sum/2
  Sum/1 -> M22/1  "a+2bCos(x3)"
  x3/1 -> Trigonometric Function/1

== system dPendDisEKF/EKFDis/Predictor/F(x)/M matrix/M2/M24 ==
  x3 : Inport
  Constant : Constant  Value=d  OutDataType=sfix(16)  OutScaling=2^0
  Gain1 : Gain  Gain=b  ParameterDataType=sfix(16)  ParameterScaling=2^0  OutDataType=sfix(16)  OutScaling=2^0
  Sum : Sum  OutDataType=sfix(16)  OutScaling=2^0
  Trigonometric Function : Trigonometry  Operator=cos
  M24 : Outport
  wires:
  Constant/1 -> Sum/1
  x3/1 -> Trigonometric Function/1
  Sum/1 -> M24/1  "d+bCos(x3)"
  Gain1/1 -> Sum/2
  Trigonometric Function/1 -> Gain1/1
